simulink model "Discrete_model_Kalman_Filter"  (R2021a)
settings: Solver=VariableStepAuto  StartTime=0.0  StopTime=18.0  RelTol=1e-3
values from neighbouring files (symbols this model uses):
  A = [0 0 1 0 ... (first row only)    [Support_Script.m]    (also in Support_Script_with_noise.m)
  B = [0; 0; 1/mc; 1/(L*mc)]    [Support_Script.m]    (also in Support_Script_with_noise.m)
  C = [1 0 0 0]    [Support_Script.m]    (also in Support_Script_with_noise.m)
  Q = diag([0 0 0 0.005])    [Support_Script.m]    (also in Support_Script_with_noise.m)
  R = [0.001]    [Support_Script.m]    (also in Support_Script_with_noise.m)
settings Model: Creator=jai_bhawani  LastModifiedBy=jai_bhawani

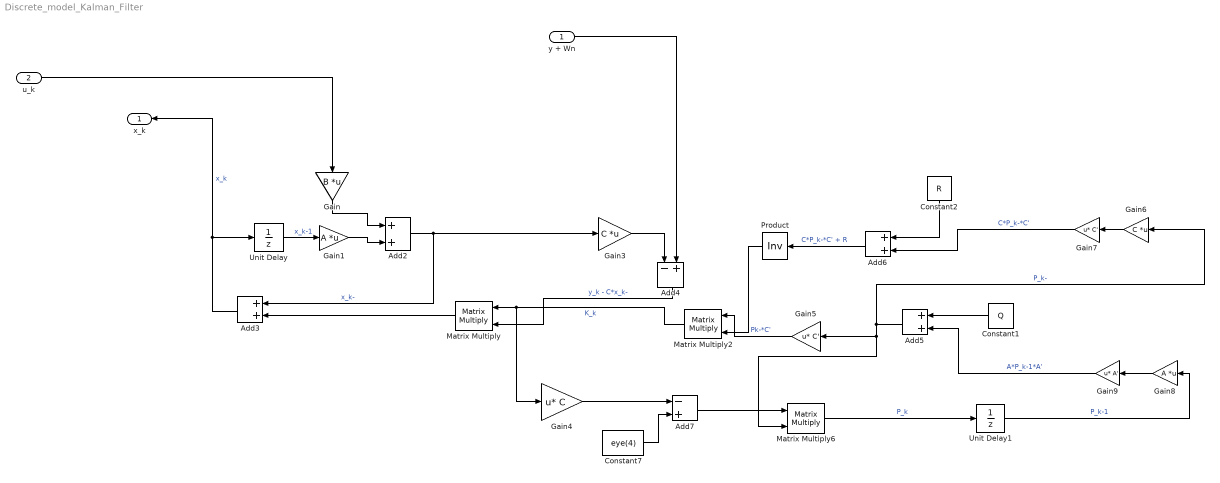
== system Discrete_model_Kalman_Filter ==
  y + Wn : Inport
  u_k : Inport  Port=2
  Add{2..3,5..6} (4 alike) : Sum
  Add4 : Sum  Inputs=-+
  Add7 : Sum  Inputs=-+
  Constant1 : Constant  Value=Q
  Constant2 : Constant  Value=R
  Constant7 : Constant  Value=eye(4)
  Gain : Gain  Gain=B  Multiplication=Matrix(K*u)
  Gain1 : Gain  Gain=A  Multiplication=Matrix(K*u)
  Gain3 : Gain  Gain=C  Multiplication=Matrix(K*u)
  Gain4 : Gain  Gain=C  Multiplication=Matrix(u*K)
  Gain5 : Gain  Gain=C'  Multiplication=Matrix(u*K)
  Gain6 : Gain  Gain=C  Multiplication=Matrix(K*u)
  Gain7 : Gain  Gain=C'  Multiplication=Matrix(u*K)
  Gain8 : Gain  Gain=A  Multiplication=Matrix(K*u)
  Gain9 : Gain  Gain=A'  Multiplication=Matrix(u*K)
  Matrix Multiply : Product  Multiplication=Matrix(*)
  Matrix Multiply2 : Product  Multiplication=Matrix(*)
  Matrix Multiply6 : Product  Multiplication=Matrix(*)
  Product : Product  Inputs=/  Multiplication=Matrix(*)
  Unit Delay : UnitDelay  SampleTime=-1  HasFrameUpgradeWarning=on
  Unit Delay1 : UnitDelay  SampleTime=-1  HasFrameUpgradeWarning=on
  x_k : Outport
  wires:
  Matrix Multiply/1 -> Add3/2
  Product/1 -> Matrix Multiply2/2
  Gain6/1 -> Gain7/1
  Add7/1 -> Matrix Multiply6/1
  u_k/1 -> Gain/1
  Gain7/1 -> Add6/2  "C*P_k-*C'"
  Gain4/1 -> Add7/1
  Constant7/1 -> Add7/2
  Gain1/1 -> Add2/2
  Gain3/1 -> Add4/1
  Constant2/1 -> Add6/1
  Gain8/1 -> Gain9/1
  Matrix Multiply2/1 -> Gain4/1, Matrix Multiply/1  "K_k"
  Matrix Multiply6/1 -> Unit Delay1/1  "P_k"
  y + Wn/1 -> Add4/2
  Gain5/1 -> Matrix Multiply2/1  "Pk-*C'"
  Gain/1 -> Add2/1
  Add5/1 -> Gain6/1, Matrix Multiply6/2, Gain5/1  "P_k-"
  Unit Delay1/1 -> Gain8/1  "P_k-1"
  Add6/1 -> Product/1  "C*P_k-*C' + R"
  Add3/1 -> x_k/1, Unit Delay/1  "x_k"
  Constant1/1 -> Add5/1
  Gain9/1 -> Add5/2  "A*P_k-1*A'"
  Unit Delay/1 -> Gain1/1  "x_k-1"
  Add4/1 -> Matrix Multiply/2  "y_k - C*x_k-"
  Add2/1 -> Gain3/1, Add3/1  "x_k-"
